simulink model "buck_dbl_cross_yt"  (R2021b)
settings: Solver=ode15s  StartTime=0.0  StopTime=400e-3  MaxStep=1e-7  RelTol=1e-3
undefined symbols (not defined in the file): dspblkcrossspectrumtfe
libraries: fl_lib x5, ee_lib x4, nesl_utility x3, dsparch4 x3, dspsrcs4 x2, slpidlib x1, simulink_extras x1, dspspect3 x1, dspmathops x1
settings Model: FPTShortcutValueString='{{},{''BaselineRun'',1,1,1,''BaselineRun'','''',{},''M'','''',''''},{''BaselineRun_2'',1,1,1,''BaselineRun_2'','''',{},''M'',''D'',''''}}'  SimulationMode=accelerator  NumberOfSteps=100  Creator=kschutz  LastModifiedBy=kschutz
settings SolverCC: AlgebraicLoopSolver=TrustRegion  SolverResetMethod=Robust
settings DebuggingCC: SFMachineParentedDataDiag=warning

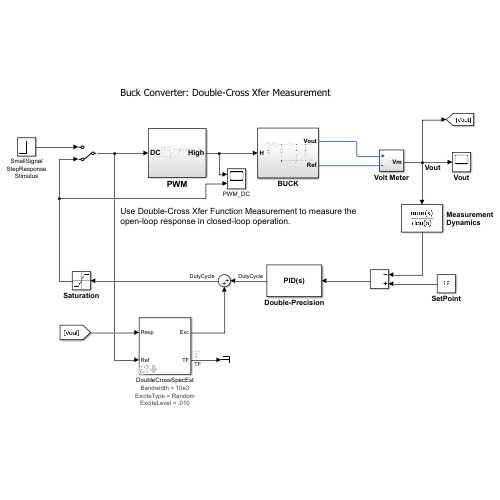
[thumbnail: Simulink's stored preview of the top-level diagram]
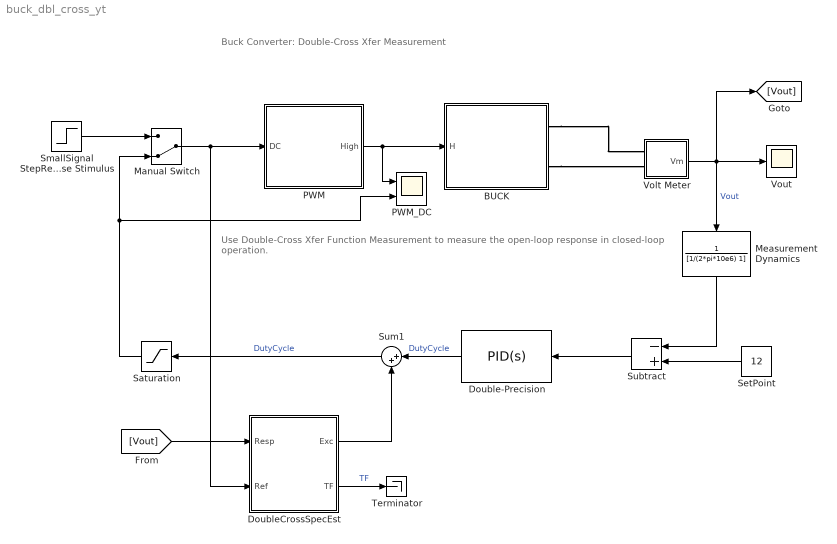
== system buck_dbl_cross_yt ==
  note: Use Double-Cross Xfer Function Measurement to measure the
      | open-loop response in closed-loop operation.
  note: Buck Converter: Double-Cross Xfer Measurement
  BUCK : Subsystem  VariantControl=BUCK_sel ==1
  Double-Precision : slpidlib/PID Controller  Controller=PID  Form=Parallel  TimeDomain=Continuous-time  UseExternalTs=off  SampleTime=1/(5*50e3)  IntegratorMethod=Forward Euler  FilterMethod=Forward Euler  ControllerParametersSource=internal  P=3  I=800  D=0  UseFilter=on  N=100  TunerSelectOption=Transfer Function Based (PID Tuner App)  InitialConditionSource=internal  InitialConditionForIntegrator=0  InitialConditionForFilter=0  DifferentiatorICPrevScaledInput=0  ExternalReset=none  TrackingMode=off  Kt=1  LimitOutput=off  SatLimitsSource=internal  UpperSaturationLimit=inf  LowerSaturationLimit=-inf  LinearizeAsGain=on  AntiWindupMode=none  Kb=1  POutMin=[]  POutMax=[]  IOutMin=[]  IOutMax=[]  DOutMin=[]  DOutMax=[]  NOutMin=[]  NOutMax=[]  SumOutMin=[]  SumOutMax=[]  SaturationOutMin=[]  SaturationOutMax=[]  PParamMin=[]  PParamMax=[]  IParamMin=[]  IParamMax=[]  DParamMin=[]  DParamMax=[]  NParamMin=[]  NParamMax=[]  KbParamMin=[]  KbParamMax=[]  KtParamMin=[]  KtParamMax=[]  KbOutMin=[]  KbOutMax=[]  KtOutMin=[]  KtOutMax=[]  IntegratorOutMin=[]  IntegratorOutMax=[]  FilterOutMin=[]  FilterOutMax=[]  SumI1OutMin=[]  SumI1OutMax=[]  SumI2OutMin=[]  SumI2OutMax=[]  SumI3OutMin=[]  SumI3OutMax=[]  SumI4OutMin=[]  SumI4OutMax=[]  SumDOutMin=[]  SumDOutMax=[]  DifferentiatorOutMin=[]  DifferentiatorOutMax=[]  FilterDiffOutCoefMin=[]  FilterDiffOutCoefMax=[]  ReciprocalOutMin=[]  ReciprocalOutMax=[]  SumDenOutMin=[]  SumDenOutMax=[]  SumNumOutMin=[]  SumNumOutMax=[]  DivideOutMin=[]  DivideOutMax=[]  UdiffTsProdOutMin=[]  UdiffTsProdOutMax=[]  NTsProdOutMin=[]  NTsProdOutMax=[]  UintegralTsProdOutMin=[]  UintegralTsProdOutMax=[]  UngainTsProdOutMin=[]  UngainTsProdOutMax=[]  IntegratorContinuousStateAttributes=''  IntegratorStateMustResolveToSignalObject=off  IntegratorRTWStateStorageClass=Auto  FilterContinuousStateAttributes=''  FilterStateMustResolveToSignalObject=off  FilterRTWStateStorageClass=Auto  ParallelPVariant=InternalParameters  IdealPVariant=Disabled  IVariant=InternalParameters  DVariant=InternalParameters  IntegratorVariant=Continuous  SatVariant=Disabled  AWVariant=Passthrough  PCopyVariant=Disabled  TRVariant=Disabled  FdbkBlocksVariant=Forward  IdealPFdbkVariant=Disabled  SatFdbkVariant=Disabled  DerivativeFilterVariant=ContFilter  NVariant=InternalParameters  NCopyVariant=Disabled  FilterICVariant=InternalICsFilter  IntegratorICVariant=InternalICs  ExternalResetVariant=Disabled  TRSumVariant=Passthrough  SumFdbkVariant=Disabled  SumVariant=Sum_PID  TsampFilterVariant=InternalTs  TsampNgainVariant=Passthrough  TsampIntegralVariant=Passthrough  ExternalSaturationOutDataTypeStr=Inherit: Same as second input
  DoubleCrossSpecEst : Subsystem  AncestorBlock=Kblocks/Analog Transfer Function Estimator  mask(Baseband Analog Transfer Function Estimator){BW=10e3, Level=.010, ExcitationType=Random, Nfft=512, Navg=10, HoldOff=30e-3}
      mask prompts: BW "Bandwidth"; Level "Excitation Level"; ExcitationType "Excitation Type"; Nfft "FFT size"; Navg "Number of Averages"; HoldOff "Hold Off (seconds)"
      mask init:
      | % Select subset of FFT bins that are not aliased
      | % for output and display purposes.
      | % Said subset is based on the oversampling factor.
      | % Here we use a 2.56x oversampling factor.
      | % For example, for a 1024 point FFT size, the relatively
      | % alias free FFT bins would be bins 1 to 401.
      | % floor(1024/2.56) + 1 = 401.
      | OSR = 2.56;
      | AliasFree = floor(Nfft/OSR) + 1;
      | %debug_init_cmd
      | sel=get_param(gcb,'ExcitationType');
      | switch sel
      |     case 'Chirp'
      |         set_param([gcb,'/Excitation_Variant'],'LabelModeActiveChoice','excitation_type==1');
      |         set_param([gcb,'/TFE/DBL_XSPEC_EST/XSPEC_EST1'],'Window','Rectangular');
      |         set_param([gcb,'/TFE/DBL_XSPEC_EST/XSPEC_EST2'],'Window','Rectangular');
      |     case 'Random'
      |         set_param([gcb,'/Excitation_Variant'],'LabelModeActiveChoice','excitation_type==2');
      |         set_param([gcb,'/TFE/DBL_XSPEC_EST/XSPEC_EST1'],'Window','Hann');
      |         set_param([gcb,'/TFE/DBL_XSPEC_EST/XSPEC_EST2'],'Window','Hann');
      |     otherwise
      |         error(['Unknown excitation type in initialization command of Double Cross-Spectrum Estimator block = ',sel]);
      | end
      settings: AttributesFormatString=|
      | Bandwidth = %<BW>
      | ExciteType = %<ExcitationType>
      | ExciteLevel = %<Level>
      mask TypeOptions ExcitationType: Chirp | Random
  Manual Switch : ManualSwitch  CurrentSetting=0
  Measurement Dynamics : TransferFcn  Denominator=[1/(2*pi*10e6) 1]
  PWM : Subsystem  VariantControl=PWM_sel==1
  PWM_DC : Scope  NumInputPorts=2
  Saturation : Saturate  UpperLimit=.97  LowerLimit=.02
  SetPoint : Constant  Value=12
  SmallSignal StepResponse Stimulus : Step  Time=10e-3  Before=.4  After=.41  SampleTime=0
  Subtract : Sum  Inputs=-+
  Sum1 : Sum  Inputs=|++
  Terminator : Terminator
  Volt Meter : Subsystem
  Vout : Scope
  wires:
  Volt Meter/1(Vm) -> [Vout], Measurement Dynamics/1, Vout/1  "Vout"
  Measurement Dynamics/1 -> Subtract/1
  SetPoint/1 -> Subtract/2
  Subtract/1 -> Double-Precision/1
  PWM/1(High) -> PWM_DC/1, BUCK/1(H)
  DoubleCrossSpecEst/2(TF) -> Terminator/1  "TF"
  SmallSignal StepResponse Stimulus/1 -> Manual Switch/1
  Saturation/1 -> Manual Switch/2, PWM_DC/2
  Manual Switch/1 -> DoubleCrossSpecEst/2(Ref), PWM/1(DC)
  [Vout] -> DoubleCrossSpecEst/1(Resp)
  DoubleCrossSpecEst/1(Exc) -> Sum1/2
  Double-Precision/1 -> Sum1/1  "DutyCycle"
  Sum1/1 -> Saturation/1  "DutyCycle"
  connections:
  BUCK/RConn1 -- Volt Meter/LConn1
  BUCK/RConn2 -- Volt Meter/LConn2

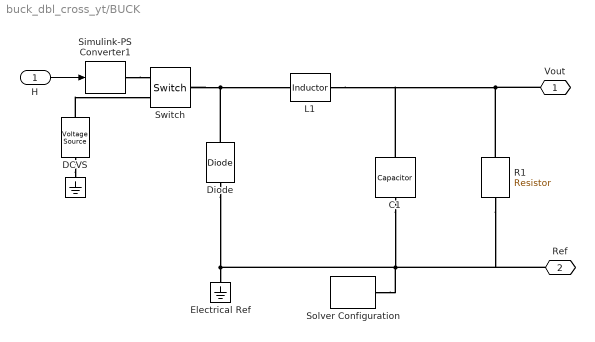
== system buck_dbl_cross_yt/BUCK ==
  H : Inport
  " " : fl_lib/Electrical/Electrical Elements/Electrical Reference
  C1 : ee_lib/Passive/Capacitor  cap_option=0  c=47e-6 F  Cvec=[1e-05, 1e-06] F  Vvec=[0, 10] V  CV_table_symmetry=1  f_vec=[1, 10] kHz  DFext_vec=[.8, 1.2]  C_tol=5  enable_C_tol=0  tol_distribution=1  nSigma=4  r=1e-6 Ohm  g=0 1/Ohm  averaging_period=0 s  enable_operating_limits=0  operating_limit_action=2  max_working_voltage_range=[-25, 25] V  power_rating=1 W  enable_faults=0  fault_action=1  Cscale_faulted=100  R_faulted=1e-3 Ohm  G_faulted=0 1/Ohm  tau_fault=1e-3 s  enable_temporal_fault=0  t_fault=1 s  enable_behavioral_fault=0  max_permissible_voltage_range=[-100, 100] V  t_fail_on_voltage=1 s  i_specify=off  i_priority=None  i=0 A  i_nominal_specify=off  i_nominal_unit=A  i_nominal_value=1  v_specify=off  v_priority=None  v=0 V  v_nominal_specify=off  v_nominal_unit=V  v_nominal_value=1  vc_specify=off  vc_priority=High  vc=0 V  vc_nominal_specify=off  vc_nominal_unit=V  vc_nominal_value=1
      settings: AttributesFormatString=%<c> %<c_unit>
  DCVS : ee_lib/Sources/Voltage Source  dc_voltage=30 V  ac_voltage=0 V  ac_shift=0 rad  ac_frequency=60 Hz  noise_mode=0  PSD=1e-9 V^2/Hz  repeatability=1  auto_seed=1073609408  user_seed=0  sample_time=1/(20*50e3) s  i_specify=off  i_priority=None  i=0 A  i_nominal_specify=off  i_nominal_unit=A  i_nominal_value=1  v_specify=off  v_priority=None  v=0 V  v_nominal_specify=off  v_nominal_unit=V  v_nominal_value=1
      settings: AttributesFormatString=%<dc_voltage> %<dc_voltage_unit>
  Diode : fl_lib/Electrical/Electrical Elements/Diode  Vf=.6 V  Ron=.001 Ohm  Goff=1e-8 1/Ohm  i_specify=off  i_priority=None  i=0 A  i_nominal_specify=off  i_nominal_unit=A  i_nominal_value=1  v_specify=off  v_priority=None  v=0 V  v_nominal_specify=off  v_nominal_unit=V  v_nominal_value=1
  Electrical Ref : fl_lib/Electrical/Electrical Elements/Electrical Reference
  L1 : ee_lib/Passive/Inductor  l=1e-3 H  L_tol=20  enable_L_tol=0  tol_distribution=1  nSigma=4  r=0 Ohm  g=1e-9 1/Ohm  enable_operating_limits=0  operating_limit_action=2  max_working_current=1 A  power_rating=1 W  enable_faults=0  fault_action=1  lambdaPercent=50  k_faulted=0.9999  turnsShort=0  openCct=0  groundShort=0  groundShortG=0 1/Ohm  tau_fault=1e-3 s  enable_temporal_fault=0  t_fault=1 s  enable_behavioral_fault=0  max_permissible_voltage=100 V  n_fail_on_voltage=1  max_permissible_current=1 A  t_fail_on_current=1 s  i_L_specify=off  i_L_priority=High  i_L=0 A  i_L_nominal_specify=off  i_L_nominal_unit=A  i_L_nominal_value=1
      settings: AttributesFormatString=%<l> %<l_unit>
  R1 : ee_lib/Passive/Resistor  R=2 Ohm  R_tol=5  enable_R_tol=0  tol_distribution=1  nSigma=4  enable_operating_limits=0  operating_limit_action=2  max_working_voltage=100 V  power_rating=1 W  enable_faults=0  fault_action=1  R_faulted=inf Ohm  enable_temporal_fault=0  t_fault=1 s  enable_behavioral_fault=0  max_permissible_current=1 A  t_fail_on_current=1 s  noise_mode=0  sample_time=1e-3 s  repeatability=1  auto_seed=4103572952  user_seed=0  Tdevice=25 degC  power_derating_T1=70 degC  power_derating_T2=155 degC  operating_temperature_range_vec=[-50, 150] degC  alpha=3.93e-3 1/K  Tmeas=25 degC  thermal_mass=100 J/K  temperature_specify=off  temperature_priority=High  temperature=298.15 K  temperature_nominal_specify=off  temperature_nominal_unit=K  temperature_nominal_value=1
      settings: AttributesFormatString=%<R> %<R_unit>
  Simulink-PS Converter1 : nesl_utility/Simulink-PS Converter  PhysicalDomain=network_engine_domain  SubClassName=ps_input  LeftPortType=input  RightPortType=output  PseudoPeriodic=off  Frequencies=[]  NoiseDistribution=none  NoiseParameters=[]  Unit=1  AffineConversion=off  FilteringAndDerivatives=provide  SimscapeFilterOrder=1  InputFilterTimeConstant=0.001  UdotUserProvided=0
      settings: SourceProductBaseCode=PW,SS
  Solver Configuration : nesl_utility/Solver Configuration  PhysicalDomain=network_engine_domain  SubClassName=solver  LeftPortType=input  RightPortType=generic  Tones=[]  Harmonics=[]  SimulateNoise=off  Profile=off  UseLocalSampling=off  EnableSwitchedLinearOptims=on  FrequencyDomain=off  UseCCode=off  RelTol=0.001  AbsTol=1e-06  MinStep=1e-09  ToWorkspace=off  RevertToSquareIcSolve=off  NumHomotopyIterations=100  PhasorMode=off  PhasorModeNumHarmonics=1  DoDC=off  ResidualTolerance=1e-09  UseLocalSolver=off  LocalSolverChoice=NE_BACKWARD_EULER_ADVANCER  LocalSolverSampleTime=0.001  DoFixedCost=off  MaxNonlinIter=3  MaxModeIter=2  ComputeImpulses=off  ImpulseIterations=2  LinearAlgebra=auto  EquationFormulation=NE_TIME_EF  DelaysMemoryBudget=1024  AutomaticFiltering=on  FilteringTimeConstant=0.001  PartitionStorageMethod=AS_NEEDED  PartitionMemoryBudget=1024  PartitionMethod=ROBUST
      settings: SourceProductBaseCode=PW,SS
  Switch : fl_lib/Electrical/Electrical Elements/Switch  R_closed=0.01 Ohm  G_open=1e-8 1/Ohm  Threshold=0.5  i_specify=off  i_priority=None  i=0 A  i_nominal_specify=off  i_nominal_unit=A  i_nominal_value=1  v_specify=off  v_priority=None  v=0 V  v_nominal_specify=off  v_nominal_unit=V  v_nominal_value=1
  Vout : PMIOPort  Side=Right
  Ref : PMIOPort  Port=2  Side=Right
  wires:
  H/1 -> Simulink-PS Converter1/1
  connections:
  Simulink-PS Converter1/RConn1 -- Switch/RConn1
  DCVS/LConn1 -- Switch/RConn2
  C1/RConn1 -- R1/RConn1 -- Ref/RConn1 -- Solver Configuration/RConn1 -- Diode/LConn1 -- Electrical Ref/LConn1
  DCVS/RConn1 -- " "/LConn1
  Vout/RConn1 -- L1/RConn1 -- C1/LConn1 -- R1/LConn1
  Diode/RConn1 -- Switch/LConn1 -- L1/LConn1

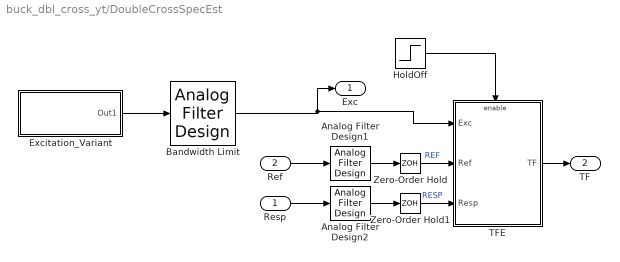
== system buck_dbl_cross_yt/DoubleCrossSpecEst ==
  Resp : Inport
  Ref : Inport  Port=2
  Analog Filter Design1 : dsparch4/Analog Filter Design  method=Elliptic  filttype=Lowpass  N=8  Wlo=2*pi*BW  Whi=80  Rp=2  Rs=100
  Analog Filter Design2 : dsparch4/Analog Filter Design  method=Elliptic  filttype=Lowpass  N=8  Wlo=2*pi*BW  Whi=80  Rp=2  Rs=100
  Bandwidth Limit : dsparch4/Analog Filter Design  method=Elliptic  filttype=Lowpass  N=8  Wlo=2*pi*BW  Whi=80  Rp=2  Rs=100
  Excitation_Variant : Subsystem  Variant=on  VariantControlMode=label  LabelModeActiveChoice=excitation_type==2
  HoldOff : Step  Time=HoldOff  SampleTime=0
  TFE : Subsystem
  Zero-Order Hold : ZeroOrderHold  SampleTime=1/(OSR*BW)
  Zero-Order Hold1 : ZeroOrderHold  SampleTime=1/(OSR*BW)
  Exc : Outport
  TF : Outport  Port=2
  wires:
  Bandwidth Limit/1 -> TFE/1(Exc), Exc/1
  HoldOff/1 -> TFE/Enable
  TFE/1(TF) -> TF/1
  Excitation_Variant/1(Out1) -> Bandwidth Limit/1
  Analog Filter Design1/1 -> Zero-Order Hold/1
  Ref/1 -> Analog Filter Design1/1
  Zero-Order Hold/1 -> TFE/2(Ref)  "REF"
  Resp/1 -> Analog Filter Design2/1
  Analog Filter Design2/1 -> Zero-Order Hold1/1
  Zero-Order Hold1/1 -> TFE/3(Resp)  "RESP"

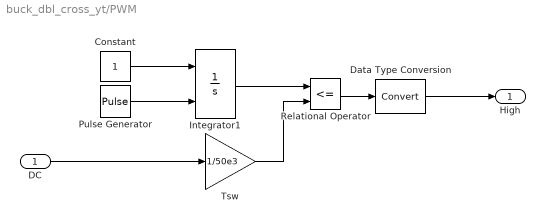
== system buck_dbl_cross_yt/PWM ==
  DC : Inport
  Constant : Constant
  Data Type Conversion : DataTypeConversion
  Integrator1 : Integrator  ExternalReset=rising  UpperSaturationLimit=1  LowerSaturationLimit=0  WrapState=on  WrappedStateLowerValue=0
  Pulse Generator : DiscretePulseGenerator  PulseType=Time based  Period=1/50e3  PulseWidth=5
  Relational Operator : RelationalOperator  Operator=<=  OutDataTypeStr=boolean  RndMeth=Simplest
  Tsw : Gain  Gain=1/50e3
  High : Outport
  wires:
  Data Type Conversion/1 -> High/1
  DC/1 -> Tsw/1
  Relational Operator/1 -> Data Type Conversion/1
  Integrator1/1 -> Relational Operator/1
  Pulse Generator/1 -> Integrator1/2
  Tsw/1 -> Relational Operator/2
  Constant/1 -> Integrator1/1

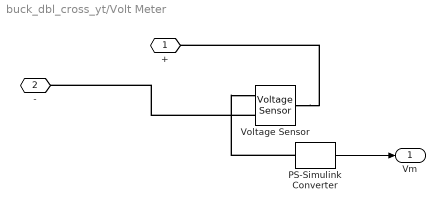
== system buck_dbl_cross_yt/Volt Meter ==
  PS-Simulink Converter : nesl_utility/PS-Simulink Converter  PhysicalDomain=network_engine_domain  SubClassName=ps_output  LeftPortType=input  RightPortType=output  PseudoPeriodic=off  Frequencies=[]  Unit=inherit  AffineConversion=off
      settings: SourceProductBaseCode=PW,SS
  Voltage Sensor : fl_lib/Electrical/Electrical Sensors/Voltage Sensor
  + : PMIOPort  Side=Left
  - : PMIOPort  Port=2  Side=Left
  Vm : Outport
  wires:
  PS-Simulink Converter/1 -> Vm/1
  connections:
  PS-Simulink Converter/LConn1 -- Voltage Sensor/RConn1
  Voltage Sensor/RConn2 -- -/RConn1
  Voltage Sensor/LConn1 -- +/RConn1

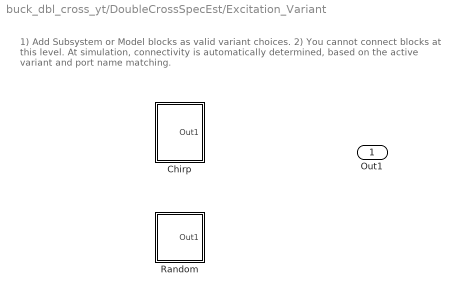
== system buck_dbl_cross_yt/DoubleCrossSpecEst/Excitation_Variant ==
  note: 1) Add Subsystem or Model blocks as valid variant choices.
      | 2) You cannot connect blocks at this level. At simulation, connectivity is automatically
      | determined, based on the active variant and port name matching.
  Chirp : Subsystem  VariantControl=excitation_type==1
  Random : Subsystem  VariantControl=excitation_type==2
  Out1 : Outport

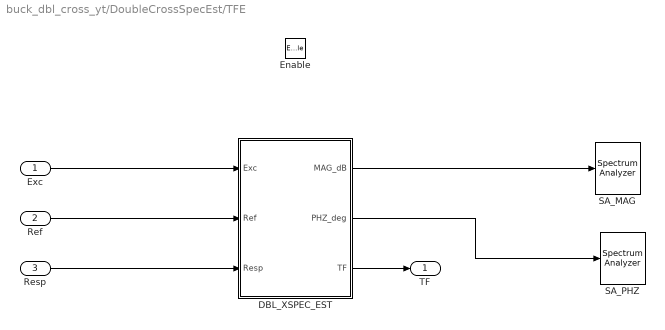
== system buck_dbl_cross_yt/DoubleCrossSpecEst/TFE ==
  Exc : Inport
  Ref : Inport  Port=2
  Resp : Inport  Port=3
  Enable : EnablePort
  DBL_XSPEC_EST : Subsystem
  SA_MAG : SpectrumAnalyzer  IsFrequencyInputMode=1
  SA_PHZ : SpectrumAnalyzer  IsFrequencyInputMode=1
  TF : Outport
  wires:
  Exc/1 -> DBL_XSPEC_EST/1(Exc)
  Ref/1 -> DBL_XSPEC_EST/2(Ref)
  Resp/1 -> DBL_XSPEC_EST/3(Resp)
  DBL_XSPEC_EST/1(MAG_dB) -> SA_MAG/1
  DBL_XSPEC_EST/2(PHZ_deg) -> SA_PHZ/1
  DBL_XSPEC_EST/3(TF) -> TF/1

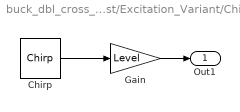
== system buck_dbl_cross_yt/DoubleCrossSpecEst/Excitation_Variant/Chirp ==
  Chirp : dspsrcs4/Chirp  sweep=Linear  mode=Unidirectional  f0=0  f1=BW  t1=Nfft/(BW*2.56)  Tsweep=Nfft/(BW*2.56)  phase=3*pi/2  Ts=1/(2.56*BW)  spf=1  datatype=Double  OutputFrames=on
  Gain : Gain  Gain=Level
  Out1 : Outport
  wires:
  Chirp/1 -> Gain/1
  Gain/1 -> Out1/1

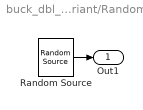
== system buck_dbl_cross_yt/DoubleCrossSpecEst/Excitation_Variant/Random ==
  Random Source : dspsrcs4/Random Source  SrcType=Uniform  NormMethod=Ziggurat  CltLength=12  MinVal=-Level  MaxVal=Level  MeanVal=0  VarVal=1  RepMode=Specify seed  rawSeed=1  IsInherit=off  SampMode=Discrete  SampTime=1/(2.56*BW)  SampFrame=1  DataType=Double  OutComplex=Real  OutputFrames=off
  Out1 : Outport
  wires:
  Random Source/1 -> Out1/1

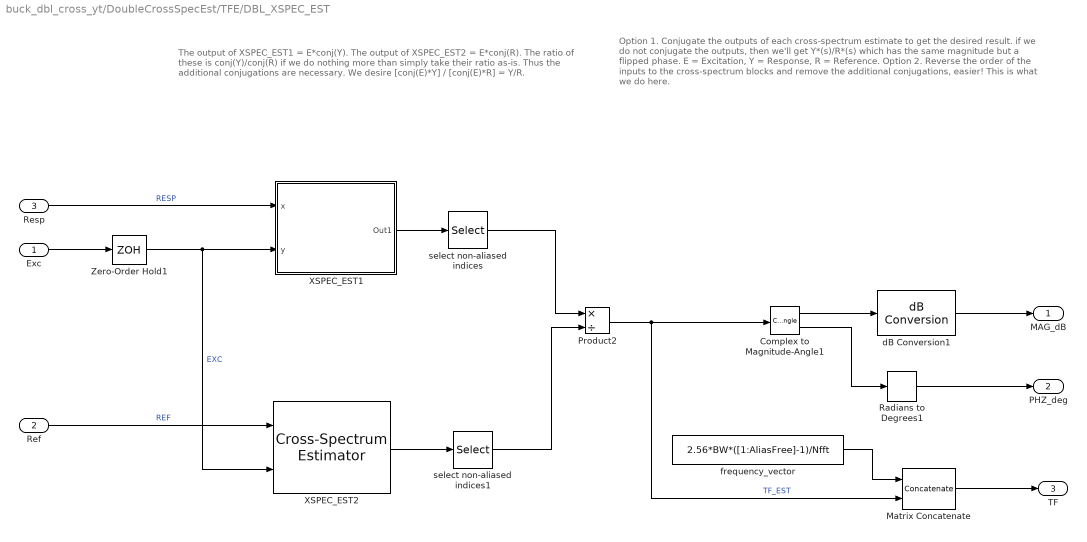
== system buck_dbl_cross_yt/DoubleCrossSpecEst/TFE/DBL_XSPEC_EST ==
  note: The output of XSPEC_EST1 = E*conj(Y).
      | The output of XSPEC_EST2 = E*conj(R).
      | The ratio of these is conj(Y)/conj(R) if we do nothing more than
      | simply take their ratio as-is. Thus the additional conjugations
      | are necessary.
      | We desire [conj(E)*Y] / [conj(E)*R] = Y/R.
  note: Option 1. Conjugate the outputs of each cross-spectrum estimate to get the desired result. if we do not conjugate the outputs, then we'll get Y*(s)/R*(s) which has the same magnitude but a flipped phase. E = Excitation, Y = Response, R = Reference.
      |
      | Option 2. Reverse the order of the inputs to the cross-spectrum blocks and remove the additional conjugations, easier!
      | This is what we do here.
  Exc : Inport
  Ref : Inport  Port=2
  Resp : Inport  Port=3
  Complex to Magnitude-Angle1 : ComplexToMagnitudeAngle
  Matrix Concatenate : Concatenate  Mode=Multidimensional array  ConcatenateDimension=2
  Product2 : Product  Inputs=*/  InputSameDT=on  SaturateOnIntegerOverflow=on  OutDataTypeStr=Inherit: Same as first input
  Radians to Degrees1 : simulink_extras/Transformations/Radians to Degrees
  XSPEC_EST1 : Subsystem  InitFcn=dspblkcrossspectrumtfe(gcb,'setup')  TreatAsAtomicUnit=on  mask(Cross-Spectrum Estimator){WindowMode=Specify on dialog, WindowLength=Nfft, Overlap=0, AveragingMethod=Running, ForgettingFactorPort=off, ForgettingFactor=0.9, SpectralAverages=Navg, FFTLengthSource=Property, FFTLength=Nfft, Window=Hann, SidelobeAttenuation=60, FrequencyRange=One-sided, InheritSampleRate=on, SampleRate=44100, SimulateUsing=Interpreted execution}
      mask prompts: WindowMode "dsp:SpectrumEstimation_BlockDialog:WindowMode_MP"; WindowLength "dsp:SpectrumEstimation_BlockDialog:WindowLength_MP"; Overlap "dsp:SpectrumEstimation_BlockDialog:Overlap_MP"; AveragingMethod "dsp:SpectrumEstimation_BlockDialog:AveragingMethod_MP"; ForgettingFactorPort "Specify forgetting factor from input port"; ForgettingFactor "Forgetting factor:"; SpectralAverages "dsp:SpectrumEstimation_BlockDialog:SpectralAverages_MP"; FFTLengthSource "dsp:SpectrumEstimation_BlockDialog:FFTLengthSource_MP"; FFTLength "dsp:SpectrumEstimation_BlockDialog:FFTLength_MP"; Window "dsp:SpectrumEstimation_BlockDialog:Window_MP"; SidelobeAttenuation "dsp:SpectrumEstimation_BlockDialog:SidelobeAttenuation_MP"; FrequencyRange "dsp:SpectrumEstimation_BlockDialog:FrequencyRange_MP"; InheritSampleRate "dsp:SpectrumEstimation_BlockDialog:InheritSampleRate_MP"; SampleRate "dsp:SpectrumEstimation_BlockDialog:SampleRate_MP"; SimulateUsing "dsp:SpectrumEstimation_BlockDialog:SimulateUsing_MP"
      mask help: dsp:SpectrumEstimation_BlockDialog:CrossSpectrumEstimator_MaskDesc
      mask init:
      | dspblkcrossspectrumtfe(gcb,'init');
      settings: AttributesFormatString=Window = %<Window>
      mask Help: eval('blocksethelp');
      mask TypeOptions WindowMode: dsp:SpectrumEstimation_BlockDialog:WindowLengthSourceEnum_SameAsInput | dsp:SpectrumEstimation_BlockDialog:WindowLengthSourceEnum_Dialog
      mask Callback WindowMode: dspblkcrossspectrumtfe(gcb,'dynamic','WindowMode')
      mask TypeOptions AveragingMethod: dsp:SpectrumEstimation_BlockDialog:AveragingMethodEnum_Running | dsp:SpectrumEstimation_BlockDialog:AveragingMethodEnum_Exponential
      mask Callback AveragingMethod: dspblkcrossspectrumtfe(gcb,'dynamic','AveragingMethod')
      mask TypeOptions ForgettingFactorPort: Cross-Spectrum Estimator/ForgettingFactorPort
      mask Callback ForgettingFactorPort: dspblkcrossspectrumtfe(gcb,'dynamic','ForgettingFactorPort')
      mask TypeOptions ForgettingFactor: Cross-Spectrum Estimator/ForgettingFactor
      mask TypeOptions FFTLengthSource: dsp:SpectrumEstimation_BlockDialog:Auto | dsp:SpectrumEstimation_BlockDialog:Property
      mask Callback FFTLengthSource: dspblkcrossspectrumtfe(gcb,'dynamic','FFTLengthSource')
      mask TypeOptions Window: dsp:SpectrumEstimation_BlockDialog:WindowEnum_Chebyshev | dsp:SpectrumEstimation_BlockDialog:WindowEnum_FlatTop | dsp:SpectrumEstimation_BlockDialog:WindowEnum_Hamming | dsp:SpectrumEstimation_BlockDialog:WindowEnum_Hann | dsp:SpectrumEstimation_BlockDialog:WindowEnum_Kaiser | dsp:SpectrumEstimation_BlockDialog:WindowEnum_Rectangular
      mask Callback Window: dspblkcrossspectrumtfe(gcb,'dynamic','Window')
      mask TypeOptions FrequencyRange: dsp:SpectrumEstimation_BlockDialog:FrequencyRangeEnum_OneSided | dsp:SpectrumEstimation_BlockDialog:FrequencyRangeEnum_TwoSided | dsp:SpectrumEstimation_BlockDialog:FrequencyRangeEnum_Centered
      mask Callback InheritSampleRate: dspblkcrossspectrumtfe(gcb,'dynamic','InheritSampleRate')
      mask TypeOptions SimulateUsing: dsp:SpectrumEstimation_BlockDialog:SimulateUsingEnum_CG | dsp:SpectrumEstimation_BlockDialog:SimulateUsingEnum_Interpreted
      mask DialogControl WindowMode Prompt: Window length source:
      mask DialogControl WindowLength Prompt: Window length:
      mask DialogControl Overlap Prompt: Window overlap (%):
      mask DialogControl AveragingMethod Prompt: Averaging method:
      mask DialogControl SpectralAverages Prompt: Number of spectral averages:
      mask DialogControl FFTLengthSource Prompt: FFT length source:
      mask DialogControl FFTLength Prompt: FFT length:
      mask DialogControl Window Prompt: Window function:
      mask DialogControl SidelobeAttenuation Prompt: Sidelobe attenuation of window (dB):
      mask DialogControl FrequencyRange Prompt: Frequency range:
      mask DialogControl InheritSampleRate Prompt: Inherit sample rate from input
      mask DialogControl SampleRate Prompt: Sample rate (Hz):
      mask DialogControl SimulateUsing Prompt: Simulate using
      mask Display:
      | fprintf(getString(message('dsp:system:SpectrumEstimatorBase:CrossSpectrumEstimatorIcon')))
      | blk = gcbh;
      | port_label('input', 1, 'x')
      | port_label('input', 2, 'y')
      | if strcmp(get_param(blk,'ForgettingFactorPort'),'on')
      |   port_label('input', 3, 'lambda');
      | end
  XSPEC_EST2 : dspspect3/Cross-Spectrum Estimator  WindowMode=Specify on dialog  WindowLength=Nfft  Overlap=0  AveragingMethod=Running  ForgettingFactorPort=off  ForgettingFactor=0.9  SpectralAverages=Navg  FFTLengthSource=Property  FFTLength=Nfft  Window=Hann  SidelobeAttenuation=60  FrequencyRange=One-sided  InheritSampleRate=on  SampleRate=44100  SimulateUsing=Interpreted execution
      settings: AttributesFormatString=Window = %<Window>  SourceProductBaseCode=DS
  Zero-Order Hold1 : ZeroOrderHold  SampleTime=1/(OSR*BW)
  dB Conversion1 : dspmathops/dB Conversion  dBtype=dB  intype=Amplitude  R=1  fuzz=off
  frequency_vector : Constant  Value=2.56*BW*([1:AliasFree]-1)/Nfft
  select non-aliased indices : Selector  NumberOfDimensions=2  InputPortWidth=3  IndexOptions=Index vector (dialog),Select all  Indices=[1:AliasFree ],1  OutputSizes=1,1
  select non-aliased indices1 : Selector  NumberOfDimensions=2  InputPortWidth=3  IndexOptions=Index vector (dialog),Select all  Indices=[1:AliasFree ],1  OutputSizes=1,1
  MAG_dB : Outport
  PHZ_deg : Outport  Port=2
  TF : Outport  Port=3
  wires:
  Exc/1 -> Zero-Order Hold1/1
  XSPEC_EST1/1(Out1) -> select non-aliased indices/1
  XSPEC_EST2/1 -> select non-aliased indices1/1
  Complex to Magnitude-Angle1/2 -> Radians to Degrees1/1
  dB Conversion1/1 -> MAG_dB/1
  Complex to Magnitude-Angle1/1 -> dB Conversion1/1
  Product2/1 -> Complex to Magnitude-Angle1/1, Matrix Concatenate/2  "TF_EST"
  Zero-Order Hold1/1 -> XSPEC_EST2/2, XSPEC_EST1/2(y)  "EXC"
  Radians to Degrees1/1 -> PHZ_deg/1
  Matrix Concatenate/1 -> TF/1
  frequency_vector/1 -> Matrix Concatenate/1
  select non-aliased indices1/1 -> Product2/2
  select non-aliased indices/1 -> Product2/1
  Resp/1 -> XSPEC_EST1/1(x)  "RESP"
  Ref/1 -> XSPEC_EST2/1  "REF"

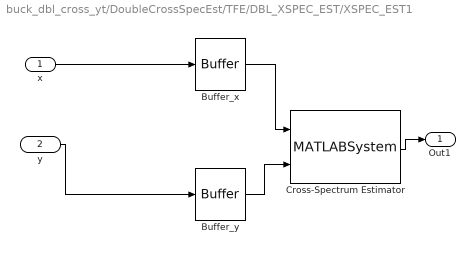
== system buck_dbl_cross_yt/DoubleCrossSpecEst/TFE/DBL_XSPEC_EST/XSPEC_EST1 ==
  x : Inport
  y : Inport  Port=2
  Buffer_x : Buffer  N=WindowLength  OutputFrames=off
  Buffer_y : Buffer  N=WindowLength  OutputFrames=off
  Cross-Spectrum Estimator : MATLABSystem  System=dsp.simulink.CrossSpectrumEstimator  AveragingMethod=Running  SpectralAverages=10  ForgettingFactorPort=off  ForgettingFactor=ForgettingFactor  FFTLengthSource=Property  FFTLength=512  Window=Hann  SidelobeAttenuation=60  FrequencyRange=onesided  InheritSampleRate=on  SampleRate=1  SimulateUsing=Interpreted execution
      mask Type: dsp.simulink.CrossSpectrumEstimator
      mask Display:
      | disp(['Cross-Spectrum' char(10) 'Estimator']);
      | port_label('input',1,'x');
      | port_label('input',2,'y');
  Out1 : Outport  VectorParamsAs1DForOutWhenUnconnected=off
  wires:
  x/1 -> Buffer_x/1
  Buffer_x/1 -> Cross-Spectrum Estimator/1
  Buffer_y/1 -> Cross-Spectrum Estimator/2
  y/1 -> Buffer_y/1
  Cross-Spectrum Estimator/1 -> Out1/1
